simulink model "building_HVAC_V00_027_AI_2019b"  (R2021b)
settings: Solver=ode3  StartTime=1425600  StopTime=1429297  FixedStep=0.1  RelTol=1e-3
model workspace (MAT data in the model file):
  A = 0
  pystep = 1
values from neighbouring files (symbols this model uses):
  Air_Cp = [1007 1007 1006 1006 1006 1006 1006 1006 1006 1006 1007 1007 ... (21 elements, 21x1)]    [data_07.mat]    (also in data_08.mat)
  Air_density = [1.783 1.582 1.422 1.367 1.341 1.316 1.292 1.268 1.246 1.225 1.204 1.184 ... (32 elements, 32x1)]    [data_07.mat]    (also in data_08.mat)
  Air_dynamic_viscosity_PaS = [1.318e-05 1.456e-05 1.588e-05 1.64e-05 1.665e-05 1.69e-05 1.715e-05 1.74e-05 1.764e-05 1.789e-05 1.813e-05 1.837e-05 ... (32 elements, 32x1)]    [data_07.mat]    (also in data_08.mat)
  Air_enthalpy = [325420 335490 345550 355620 365680 375730 385790 395850 405910 415970 426040 436110 ... (21 elements, 21x1)]    [data_07.mat]    (also in data_08.mat)
  Air_prandtl_number = [0.734 0.72 0.711 0.707 0.705 0.701 0.699 0.698 0.699 0.702]    [data_07.mat]    (also in data_08.mat)
  Air_Temp_for_Cp = [200 210 220 230 240 250 260 270 280 290 300 310 ... (21 elements, 21x1)]    [data_07.mat]    (also in data_08.mat)
  Air_Temp_for_density = [-75 -50 -25 -15 -10 -5 0 5 10 15 20 25 ... (32 elements, 32x1)]    [data_07.mat]    (also in data_08.mat)
  Air_Temp_for_dynamic_viscosity = [-75 -50 -25 -15 -10 -5 0 5 10 15 20 25 ... (32 elements, 32x1)]    [data_07.mat]    (also in data_08.mat)
  Air_Temp_for_enthalpy = [200 210 220 230 240 250 260 270 280 290 300 310 ... (21 elements, 21x1)]    [data_07.mat]    (also in data_08.mat)
  Air_Temp_for_prandtl_number = [-100 -50 0 25 50 100 150 200 250 300]    [data_07.mat]    (also in data_08.mat)
  Air_Temp_for_thermal_conductivity = [-190 -150 -100 -75 -50 -25 -15 -10 -5 0 5 10 ... (35 elements, 35x1)]    [data_07.mat]    (also in data_08.mat)
  Air_thermal_conductivity = [0.00782 0.01169 0.0162 0.01834 0.02041 0.02241 0.0232 0.02359 0.02397 0.02436 0.02474 0.02512 ... (35 elements, 35x1)]    [data_07.mat]    (also in data_08.mat)
  Ambient_Solar_heat_Seoul_20200701_to_20200731 = [0 0 0 0 0 0 2.777777778 38.88888889 72.22222222 97.22222222 333.3333333 263.8888889 ... (745 elements, 745x1)]    [data_07.mat]    (also in data_08.mat)
  Ambient_Solar_heat_Seoul_20200701_to_20210630 = [0 0 0 0 0 2.777777778 38.88888889 72.22222222 97.22222222 333.3333333 263.8888889 152.7777778 ... (8736 elements, 8736x1)]    [data_07.mat]    (also in data_08.mat)
  Ambient_Solar_heat_Seoul_20200801_to_20200831 = [0 0 0 0 0 0 2.777777778 11.11111111 38.88888889 63.88888889 127.7777778 258.3333333 ... (745 elements, 745x1)]    [data_07.mat]    (also in data_08.mat)
  Ambient_Solar_heat_Seoul_20200901_to_20200930 = [0 0 0 0 0 0 0 22.22222222 108.3333333 141.6666667 211.1111111 386.1111111 ... (721 elements, 721x1)]    [data_07.mat]    (also in data_08.mat)
  Ambient_Temp_Seoul_20200701_to_20200731 = [18.8 18.8 18.7 18.4 18.2 18.2 18.3 18.5 19.1 19.6 21.2 21.6 ... (745 elements, 745x1)]    [data_07.mat]    (also in data_08.mat)
  Ambient_Temp_Seoul_20200701_to_20210630 = [18.8 18.7 18.4 18.2 18.2 18.3 18.5 19.1 19.6 21.2 21.6 21.7 ... (8736 elements, 8736x1)]    [data_07.mat]    (also in data_08.mat)
  Ambient_Temp_Seoul_20200801_to_20200831 = [25 24.6 24.6 24.7 24.7 24.5 24.3 24.3 24.6 25 25.7 26.8 ... (745 elements, 745x1)]    [data_07.mat]    (also in data_08.mat)
  Ambient_Temp_Seoul_20200901_to_20200930 = [26.2 25.8 25.5 24.9 24.5 24.3 24 23.9 24.4 24.8 25.7 26.6 ... (721 elements, 721x1)]    [data_07.mat]    (also in data_08.mat)
  Ambient_Time_Seoul_20200701_to_20200731 = [0 3600 7200 10800 14400 18000 21600 25200 28800 32400 36000 39600 ... (745 elements, 745x1)]    [data_07.mat]    (also in data_08.mat)
  Ambient_Time_Seoul_20200701_to_20210630 = [0 3600 7200 10800 14400 18000 21600 25200 28800 32400 36000 39600 ... (8736 elements, 8736x1)]    [data_07.mat]    (also in data_08.mat)
  Ambient_Time_Seoul_20200901_to_20200930 = [0 3600 7200 10800 14400 18000 21600 25200 28800 32400 36000 39600 ... (721 elements, 721x1)]    [data_07.mat]    (also in data_08.mat)
  Ambient_Water_Vapor_Pressure_Seoul_20200701_to_20200731 = [18.4 18.8 18.6 18.2 17.9 17.7 18.6 18.6 18.5 19.1 19.9 19.5 ... (745 elements, 745x1)]    [data_07.mat]    (also in data_08.mat)
  Ambient_Water_Vapor_Pressure_Seoul_20200701_to_20210630 = [18.8 18.6 18.2 17.9 17.7 18.6 18.6 18.5 19.1 19.9 19.5 19.4 ... (8736 elements, 8736x1)]    [data_07.mat]    (also in data_08.mat)
  Ambient_Water_Vapor_Pressure_Seoul_20200801_to_20200831 = [28.4 27.7 28.1 28.8 29.1 28.8 28.8 29.1 29.7 30 31.3 29.8 ... (745 elements, 745x1)]    [data_07.mat]    (also in data_08.mat)
  Ambient_Water_Vapor_Pressure_Seoul_20200901_to_20200930 = [26.1 25.8 25.6 24.7 24 24.3 22.9 23.1 23.1 22.8 24 24.3 ... (721 elements, 721x1)]    [data_07.mat]    (also in data_08.mat)
  Ambient_wind_speed_Seoul_20200701_to_20200731 = [3.7 3 3 2.3 1.2 1.5 3.1 1.4 1 1.4 2.5 2.1 ... (745 elements, 745x1)]    [data_07.mat]    (also in data_08.mat)
  Ambient_wind_speed_Seoul_20200701_to_20210630 = [3 3 2.3 1.2 1.5 3.1 1.4 1 1.4 2.5 2.1 2 ... (8736 elements, 8736x1)]    [data_07.mat]    (also in data_08.mat)
  Ambient_wind_speed_Seoul_20200801_to_20200831 = [3.4 0.5 0.5 1.2 0.8 1.3 1.8 1.4 1.2 1.1 1.8 3.4 ... (745 elements, 745x1)]    [data_07.mat]    (also in data_08.mat)
  Ambient_wind_speed_Seoul_20200901_to_20200930 = [2.3 2.2 2.5 2.6 2.4 2.1 1.7 2.7 2.6 2.5 1.5 1.8 ... (721 elements, 721x1)]    [data_07.mat]    (also in data_08.mat)
  init_time = start_time +60    [SIMULINK_RUn.m]    (also in data_07.mat = 0; data_08.mat = 1425660)
  Initial_Temp = 273 + 28    (= 301)    [SIMULINK_RUn.m]    (also in data_07.mat = 285; data_08.mat = 302)
  Shadow_20200701_to_20210630 = [285 300 315 330 345 360 15 30 45 60 75 90 ... (8736 elements, 8736x1)]    [data_07.mat]    (also in data_08.mat)
  start_time = 12 * 3600 + da * day_to_sec    [SIMULINK_RUn.m]    (also in data_07.mat = 0; data_08.mat = 1425600)
  Under_30cm_ground_Temp_Seoul_20200701_to_20200731 = [22.6 22.6 22.5 22.5 22.4 22.3 22.3 22.2 22.1 22.1 22 22 ... (745 elements, 745x1)]    [data_07.mat]    (also in data_08.mat)
  Under_30cm_ground_Temp_Seoul_20200701_to_20210630 = [22.6 22.5 22.5 22.4 22.3 22.3 22.2 22.1 22.1 22 22 22 ... (8736 elements, 8736x1)]    [data_07.mat]    (also in data_08.mat)
  Under_30cm_ground_Temp_Seoul_20200801_to_20200831 = [25.6 25.6 25.6 25.5 25.5 25.5 25.4 25.4 25.3 25.3 25.3 25.2 ... (745 elements, 745x1)]    [data_07.mat]    (also in data_08.mat)
  Under_30cm_ground_Temp_Seoul_20200901_to_20200930 = [27.4 27.4 27.4 27.4 27.3 27.3 27.3 27.2 27.2 27.1 27 27 ... (721 elements, 721x1)]    [data_07.mat]    (also in data_08.mat)
  water_saturation_enthalpy_latent = [2500899.39 2498955.8 2496540.3 2494128 2491818 2489411 2487006 2484604 2482303 2479905 2477508 2475213 ... (64 elements, 64x1)]    [data_07.mat]    (also in data_08.mat)
  water_saturation_enthalpy_vapor = [2500900 2502500 2504300 2506100 2508000 2509800 2511600 2513400 2515300 2517100 2518900 2520800 ... (64 elements, 64x1)]    [data_07.mat]    (also in data_08.mat)
  water_saturation_pressure = [611.65 650.03 698.46 750.07 805.02 863.5 925.7 991.83 1062.2 1136.8 1216 1300 ... (64 elements, 64x1)]    [data_07.mat]    (also in data_08.mat)
  water_Temp_for_saturation_enthalpy_latent = [273.16 274 275 276 277 278 279 280 281 282 283 284 ... (64 elements, 64x1)]    [data_07.mat]    (also in data_08.mat)
  water_Temp_for_saturation_enthalpy_vapor = [273.16 274 275 276 277 278 279 280 281 282 283 284 ... (64 elements, 64x1)]    [data_07.mat]    (also in data_08.mat)
  water_Temp_for_saturation_pressure = [273.16 274 275 276 277 278 279 280 281 282 283 284 ... (64 elements, 64x1)]    [data_07.mat]    (also in data_08.mat)
undefined symbols (not defined in the file or in its folder): DiscIntNeverNeededParam
libraries: fuzblock x1
(part 1 of 3)
settings Model: SimulationMode=accelerator  Creator=HYUNJONG OH  LastModifiedBy=b811043
settings SolverCC: AlgebraicLoopSolver=TrustRegion  AutoInsertRateTranBlk=on
settings DataIOCC: ExternalInput=[0,input_total(1),input_total(2),input_total(3),input_total(4),input_total(5),input_total(6);(24*3600),input_total(1),input_total(2),input_total(3),input_total(4),input_total(5),input_total(6)]  SaveFormat=Array  SaveOutput=off  SaveTime=off
settings DebuggingCC: AlgebraicLoopMsg=none  SFMachineParentedDataDiag=warning  ArithmeticOperatorsInVariantConditions=warning
settings SFSimCC: CustomCodeUndefinedFunction=UseInterfaceOnly

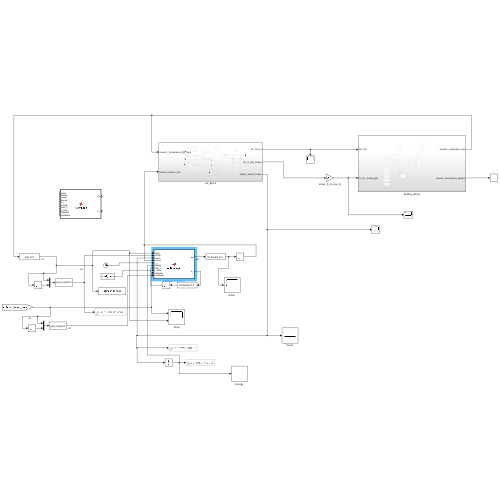
[thumbnail: Simulink's stored preview of the top-level diagram]
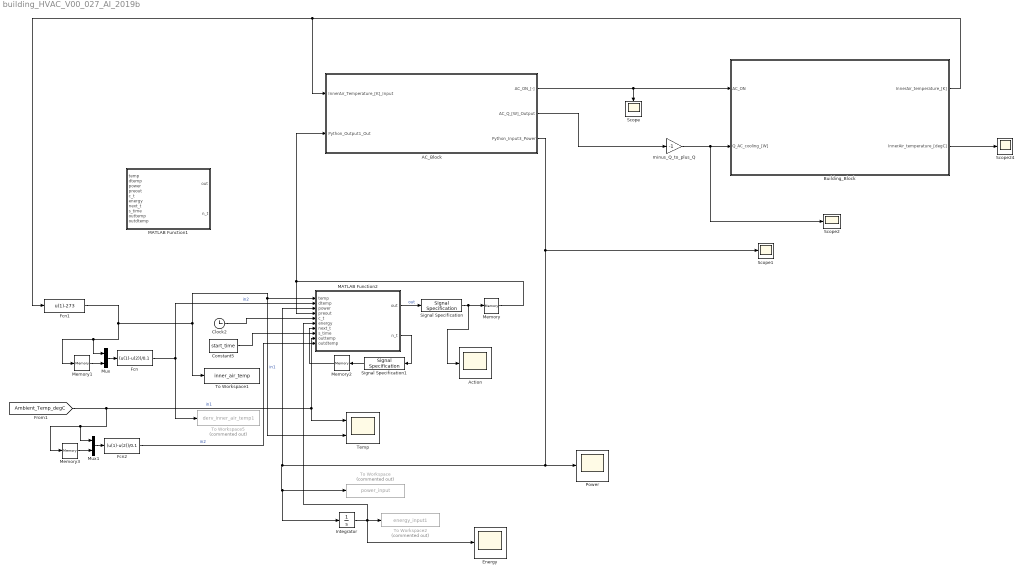
== system building_HVAC_V00_027_AI_2019b ==
  AC_Block : Subsystem
  Action : Scope
  Building_Block : Subsystem
  Clock2 : Clock
  Constant5 : Constant  Value=start_time
  Energy : Scope
  Fcn : Fcn  Expr=(u(1)-u(2))/0.1
  Fcn1 : Fcn  Expr=u(1)-273
  Fcn2 : Fcn  Expr=(u(1)-u(2))/0.1
  Integrator : Integrator
  MATLAB Function1 : MATLAB Function
  MATLAB Function2 : MATLAB Function
  Memory : Memory  InheritSampleTime=on
  Memory1 : Memory  InitialCondition=301 - 273  InheritSampleTime=on
  Memory2 : Memory  InitialCondition=init_time  InheritSampleTime=on
  Memory3 : Memory  InitialCondition=301 - 273  InheritSampleTime=on
  Mux : Mux  Inputs=2
  Mux1 : Mux  Inputs=2
  Power : Scope
  Scope{,1..2,24} (4 alike) : Scope
  Signal Specification : SignalSpecification  OutDataTypeStr=double  Dimensions=1
  Signal Specification1 : SignalSpecification  OutDataTypeStr=double  Dimensions=1
  Temp : Scope  NumInputPorts=2
  To Workspace : ToWorkspace  Commented=on  VariableName=power_input  SampleTime=-1
      settings: Save2DSignal=2-D array (concatenate along first dimension)
  To Workspace1 : ToWorkspace  VariableName=inner_air_temp  SampleTime=-1
      settings: Decimation=10  Save2DSignal=2-D array (concatenate along first dimension)
  To Workspace2 : ToWorkspace  Commented=on  VariableName=energy_input1  SampleTime=-1
      settings: Save2DSignal=2-D array (concatenate along first dimension)
  To Workspace5 : ToWorkspace  Commented=on  VariableName=derv_inner_air_temp1  SampleTime=-1
      settings: Save2DSignal=2-D array (concatenate along first dimension)
  minus_Q_to_plus_Q : Gain  Gain=-1
  wires:
  Fcn1/1 -> Memory1/1, Mux/1, MATLAB Function2/1(temp), Temp/2, To Workspace1/1  "in1"
  Fcn/1 -> MATLAB Function2/2(dtemp), To Workspace5/1  "in2"
  Mux/1 -> Fcn/1
  Memory1/1 -> Mux/2
  MATLAB Function2/1(out) -> Signal Specification/1  "out"
  Clock2/1 -> MATLAB Function2/5(c_t)
  Integrator/1 -> MATLAB Function2/6(energy), To Workspace2/1, Energy/1
  MATLAB Function2/2(n_t) -> Signal Specification1/1
  Signal Specification1/1 -> Memory2/1
  Memory2/1 -> MATLAB Function2/7(next_t)
  Constant5/1 -> MATLAB Function2/8(s_time)
  Signal Specification/1 -> Memory/1, Action/1
  AC_Block/3(Python_Input3_Power) -> Scope1/1, MATLAB Function2/3(power), Integrator/1, To Workspace/1, Power/1
  AC_Block/2(AC_Q_[W]_Output) -> minus_Q_to_plus_Q/1
  AC_Block/1(AC_ON_[-]) -> Building_Block/1(AC_ON), Scope/1
  Building_Block/1(InnerAir_temperature_[K]) -> Fcn1/1, AC_Block/1(InnerAir_Temperature_[K]_Input)
  Building_Block/2(InnerAir_temperature_[degC]) -> Scope24/1
  minus_Q_to_plus_Q/1 -> Scope2/1, Building_Block/2(Q_AC_cooling_[W])
  Memory/1 -> MATLAB Function2/4(preout), AC_Block/2(Python_Output1_Out)
  Memory3/1 -> Mux1/2
  Fcn2/1 -> MATLAB Function2/10(outdtemp)  "in2"
  Mux1/1 -> Fcn2/1
  [Ambient_Temp_degC] -> Memory3/1, Mux1/1, MATLAB Function2/9(outtemp), Temp/1  "in1"

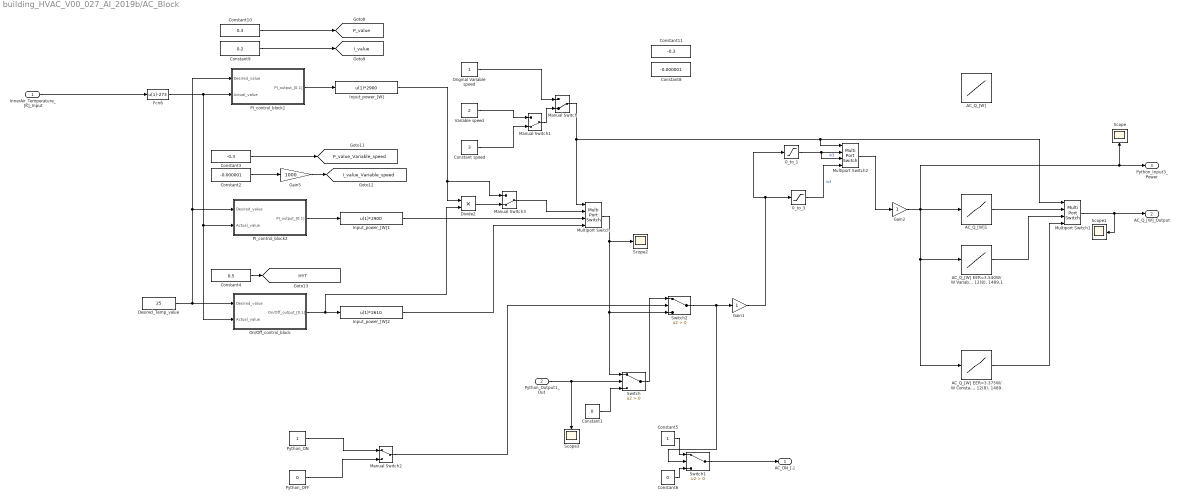
== system building_HVAC_V00_027_AI_2019b/AC_Block ==
  InnerAir_Temperature_[K]_Input : Inport
  Python_Output1_Out : Inport  Port=2
  0_to_1 : Saturate  UpperLimit=2900  LowerLimit=0
  0_to_3 : Saturate  UpperLimit=2610  LowerLimit=0
  AC_Q_[W] : Lookup_n-D  NumberOfTableDimensions=1  BreakpointsForDimension1=[0;2000]  Table=[0;((-1)*2000*3.0)]  InternalRulePriority=Speed  RndMeth=Simplest  InputSameDT=on
  "AC_Q_[W] EER=3.375W/W Constant sped type compressor is used thus, the control strategy must be ON/OFF control method Lim, J., Yoon, M. S., Al-Qahtani, T., & Nam, Y. (2019). Feasibility study on variable-speed air conditioner under hot climate based on real-scale experiment and energy simulation. Energies, 12(8), 1489." : Lookup_n-D  NumberOfTableDimensions=1  BreakpointsForDimension1=[0;2610]  Table=[0;((-1)*2610*3.375)]  InternalRulePriority=Speed  RndMeth=Simplest  InputSameDT=on
  "AC_Q_[W] EER=3.540W/W Variable sped type compressor is used thus, the control strategy should be part-load control method Lim, J., Yoon, M. S., Al-Qahtani, T., & Nam, Y. (2019). Feasibility study on variable-speed air conditioner under hot climate based on real-scale experiment and energy simulation. Energies, 12(8), 1489.1" : Lookup_n-D  NumberOfTableDimensions=1  BreakpointsForDimension1=[0;2900]  Table=[0;((-1)*2900*3.540)]  InternalRulePriority=Speed  RndMeth=Simplest  InputSameDT=on
  AC_Q_[W]1 : Lookup_n-D  NumberOfTableDimensions=1  BreakpointsForDimension1=[0;2900]  Table=[0;((-1)*2900*3.7143)]  InternalRulePriority=Speed  RndMeth=Simplest  InputSameDT=on
  Constant speed : Constant  Value=3
  Constant1 : Constant  Value=0
  Constant10 : Constant  Value=0.3
  Constant11 : Constant  Value=-0.3
  Constant2 : Constant  Value=-0.000001
  Constant3 : Constant  Value=-0.3
  Constant4 : Constant  Value=0.5
  Constant5 : Constant
  Constant6 : Constant  Value=0
  Constant8 : Constant  Value=-0.000001
  Constant9 : Constant  Value=0.2
  Desired_Temp_value : Constant  Value=25
  Divide2 : Product  Inputs=**
  Fcn6 : Fcn  Expr=u(1)-273
  Gain1 : Gain
  Gain2 : Gain
  Gain5 : Gain  Gain=1000
  Input_power_[W] : Fcn  Expr=u(1)*2900
  Input_power_[W]1 : Fcn  Expr=u(1)*2900
  Input_power_[W]2 : Fcn  Expr=u(1)*2610
  Manual Switch : ManualSwitch  CurrentSetting=0
  Manual Switch1 : ManualSwitch  CurrentSetting=0
  Manual Switch2 : ManualSwitch
  Manual Switch3 : ManualSwitch  CurrentSetting=0
  Multiport Switch : MultiPortSwitch
  Multiport Switch1 : MultiPortSwitch
  Multiport Switch2 : MultiPortSwitch
  On/Off_control_block : Subsystem
  Original Variable speed : Constant
  PI_control_block1 : Subsystem
  PI_control_block2 : Subsystem
  Python_OFF : Constant  Value=0
  Python_ON : Constant
  Scope{,1..3} (4 alike) : Scope
  Switch : Switch  Criteria=u2 > Threshold
  Switch1 : Switch  Criteria=u2 > Threshold
  Switch2 : Switch  Criteria=u2 > Threshold
  Variable speed : Constant  Value=2
  AC_ON_[-] : Outport
  AC_Q_[W]_Output : Outport  Port=2
  Python_Input3_Power : Outport  Port=3
  tag scope: HYT=global, I_value=global, I_value_Variable_speed=global, P_value=global, P_value_Variable_speed=global
  wires:
  Python_Output1_Out/1 -> Switch/2, Scope3/1
  Manual Switch/1 -> Multiport Switch1/1, Multiport Switch2/1, Multiport Switch/1
  Desired_Temp_value/1 -> PI_control_block1/1(Desired_value), PI_control_block2/1(Desired_value), On/Off_control_block/1(Desired_value)
  Fcn6/1 -> On/Off_control_block/2(Actual_value), PI_control_block2/2(Actual_value), PI_control_block1/2(Actual_value)
  InnerAir_Temperature_[K]_Input/1 -> Fcn6/1
  PI_control_block2/1(PI_output_[0,1]) -> Input_power_[W]1/1
  Constant1/1 -> Switch/3
  Constant4/1 -> [HYT]
  Original Variable speed/1 -> Manual Switch/1
  Manual Switch1/1 -> Manual Switch/2
  Constant speed/1 -> Manual Switch1/2
  Input_power_[W]1/1 -> Multiport Switch/3
  Input_power_[W]2/1 -> Multiport Switch/4
  Multiport Switch2/1 -> Gain2/1
  AC_Q_[W]1/1 -> Multiport Switch1/2
  0_to_1/1 -> Multiport Switch2/3, Multiport Switch2/2  "in3"
  PI_control_block1/1(PI_output_[0,1]) -> Input_power_[W]/1
  Variable speed/1 -> Manual Switch1/1
  On/Off_control_block/1(On/Off_output_[0,1]) -> Divide2/2, Input_power_[W]2/1
  0_to_3/1 -> Multiport Switch2/4  "in3"
  Gain2/1 -> AC_Q_[W]1/1, "AC_Q_[W] EER=3.375W/W Constant sped type compressor is used thus, the control strategy must be ON/OFF control method Lim, J., Yoon, M. S., Al-Qahtani, T., & Nam, Y. (2019). Feasibility study on variable-speed air conditioner under hot climate based on real-scale experiment and energy simulation. Energies, 12(8), 1489."/1, "AC_Q_[W] EER=3.540W/W Variable sped type compressor is used thus, the control strategy should be part-load control method Lim, J., Yoon, M. S., Al-Qahtani, T., & Nam, Y. (2019). Feasibility study on variable-speed air conditioner under hot climate based on real-scale experiment and energy simulation. Energies, 12(8), 1489.1"/1, Python_Input3_Power/1, Scope/1
  Multiport Switch1/1 -> Scope1/1, AC_Q_[W]_Output/1
  Constant5/1 -> Switch1/1
  Constant6/1 -> Switch1/3
  Gain1/1 -> 0_to_1/1, 0_to_3/1
  Multiport Switch/1 -> Scope2/1, Switch2/3, Switch/1
  Switch1/1 -> AC_ON_[-]/1
  Python_OFF/1 -> Manual Switch2/2
  Python_ON/1 -> Manual Switch2/1
  Manual Switch2/1 -> Switch2/2
  Switch/1 -> Switch2/1
  Switch2/1 -> Switch1/2, Gain1/1
  "AC_Q_[W] EER=3.540W/W Variable sped type compressor is used thus, the control strategy should be part-load control method Lim, J., Yoon, M. S., Al-Qahtani, T., & Nam, Y. (2019). Feasibility study on variable-speed air conditioner under hot climate based on real-scale experiment and energy simulation. Energies, 12(8), 1489.1"/1 -> Multiport Switch1/3
  "AC_Q_[W] EER=3.375W/W Constant sped type compressor is used thus, the control strategy must be ON/OFF control method Lim, J., Yoon, M. S., Al-Qahtani, T., & Nam, Y. (2019). Feasibility study on variable-speed air conditioner under hot climate based on real-scale experiment and energy simulation. Energies, 12(8), 1489."/1 -> Multiport Switch1/4
  Constant2/1 -> Gain5/1
  Constant3/1 -> [P_value_Variable_speed]
  Gain5/1 -> [I_value_Variable_speed]
  Input_power_[W]/1 -> Manual Switch3/1, Divide2/1
  Divide2/1 -> Manual Switch3/2
  Manual Switch3/1 -> Multiport Switch/2
  Constant9/1 -> [I_value]
  Constant10/1 -> [P_value]

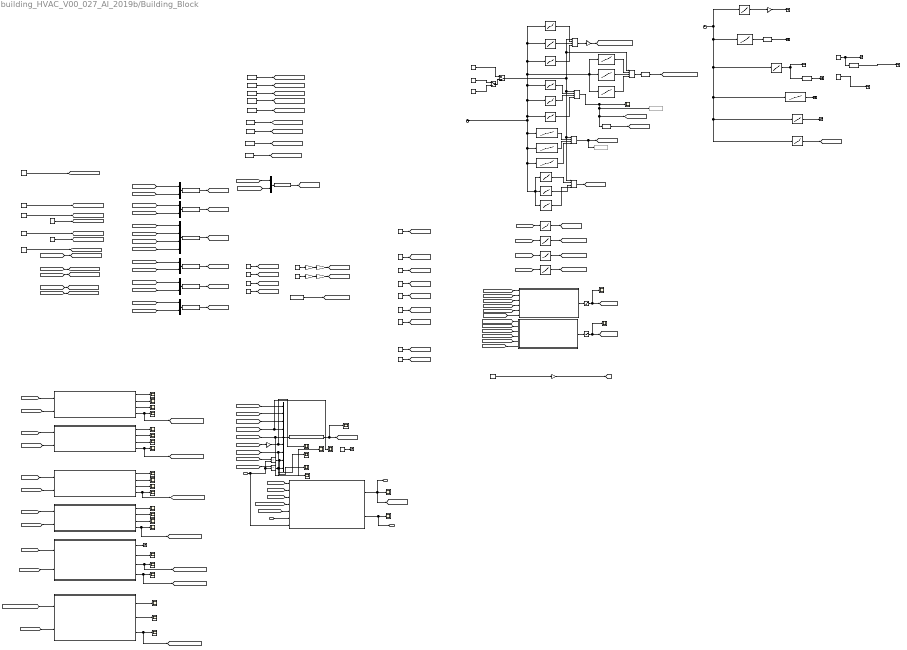
== system building_HVAC_V00_027_AI_2019b/Building_Block ==
  AC_ON : Inport
  Q_AC_cooling_[W] : Inport  Port=2
  20200701_to_20200731 : Constant
  20200801_to_20200831 : Constant  Value=2
  20200901_to_20200930 : Constant  Value=3
  A=Area_East : Fcn  Expr=u(1)*u(2)
  A=Area_North : Fcn  Expr=u(1)*u(2)
  A=Area_South - Area_Window2 : Fcn  Expr=u(1)*u(2)-u(3)*u(4)
  A=Area_West : Fcn  Expr=u(1)*u(2)
  A=Area_floor : Fcn  Expr=u(1)*u(2)
  A=Area_window : Fcn  Expr=u(1)*u(2)
  AC_blower_Volume_flow_rate_[m3/s] : Constant  Value=0.2*0.5*0.5
  AC_evaporator_vertical_length_[m] : Constant  Value=0.5
  Air_Prandtl_number_(-) _of_Air_temperature_(degC) : Lookup_n-D  NumberOfTableDimensions=1  BreakpointsForDimension1=Air_Temp_for_prandtl_number  Table=Air_prandtl_number  InternalRulePriority=Speed  RndMeth=Simplest  InputSameDT=on
  Air_Thermal_conductivity_(W/mK) _of_Air_temperature_(degC) : Lookup_n-D  NumberOfTableDimensions=1  BreakpointsForDimension1=Air_Temp_for_thermal_conductivity  Table=Air_thermal_conductivity  InternalRulePriority=Speed  RndMeth=Simplest  InputSameDT=on
  Air_density_(kg/m3) _of_Air_temperature_(degC) : Lookup_n-D  NumberOfTableDimensions=1  BreakpointsForDimension1=Air_Temp_for_density  Table=Air_density  InternalRulePriority=Speed  RndMeth=Simplest  InputSameDT=on
  Air_dynamic_viscosity_(Pa s) _of_Air_temperature_(degC) : Lookup_n-D  NumberOfTableDimensions=1  BreakpointsForDimension1=Air_Temp_for_dynamic_viscosity  Table=Air_dynamic_viscosity_PaS  InternalRulePriority=Speed  RndMeth=Simplest  InputSameDT=on
  Air_wind_speed_(m/s) _of_Air_temperature_(degC)08 : Lookup_n-D  NumberOfTableDimensions=1  BreakpointsForDimension1=Ambient_Time_Seoul_20200701_to_20200731  Table=Ambient_wind_speed_Seoul_20200801_to_20200831  InternalRulePriority=Speed  RndMeth=Simplest  InputSameDT=on
  Air_wind_speed_(m/s) _of_Air_temperature_(degC)09 : Lookup_n-D  NumberOfTableDimensions=1  BreakpointsForDimension1=Ambient_Time_Seoul_20200901_to_20200930  Table=Ambient_wind_speed_Seoul_20200901_to_20200930  InternalRulePriority=Speed  RndMeth=Simplest  InputSameDT=on
  Air_wind_speed_(m/s) _of_Air_temperature_(degC)1 : Lookup_n-D  NumberOfTableDimensions=1  BreakpointsForDimension1=Ambient_Time_Seoul_20200701_to_20210630  Table=Ambient_wind_speed_Seoul_20200701_to_20210630  InternalRulePriority=Speed  RndMeth=Simplest  InputSameDT=on
  Air_wind_speed_(m/s) _of_Time : Lookup_n-D  NumberOfTableDimensions=1  BreakpointsForDimension1=Ambient_Time_Seoul_20200701_to_20200731  Table=Ambient_wind_speed_Seoul_20200701_to_20200731  InternalRulePriority=Speed  RndMeth=Simplest  InputSameDT=on
  Ambient_Temp_K1 : Terminator
  Ambient_Temp_K2 : Terminator
  Ambient_Temp_degC1 : Terminator
  Ambient_Temp_degC2 : Terminator
  Ambient_Water_Vapor_Pressure : Terminator
  Blower_and_InnerAir_Block : Subsystem
  Clock : Clock
  Clock1 : Clock
  Constant : Constant  Value=0.1
  Constant{1..5} (5 alike) : Constant  Value=0.2
  Constant6 : Constant  Value=35
  Constant7 : Constant  Value=500
  Constant8 : Constant  Value=4500
  "Cp_cement Masonry Materials Cement mortar Frank P. Incropera and David P. DeWitt, \"Fundamentals of Heat and Mass Transfer\", (1996), FOURTH EDITION, pg. 833" : Constant  Value=780
  "Cp_insulator Board and Slab Cellular glass Frank P. Incropera and David P. DeWitt, \"Fundamentals of Heat and Mass Transfer\", (1996), FOURTH EDITION, pg. 834" : Constant  Value=1000
  Cp_window : Constant  Value=840
  East_Wall_Block : Subsystem
  East_Wall_horizontal_length_[m]3 : Constant  Value=8
  Fcn{1..5} (5 alike) : Fcn  Expr=u(1)+273
  Floorl_Block : Subsystem
  Gain : Gain
  Gain1 : Gain  Gain=0.1
  Infiltration_[L/hr] : Constant  Value=0.4
  Initial_InnerAir_Temp_[K] : Constant  Value=Initial_Temp  VectorParams1D=off
  InnerWall_Depth : Constant  Value=0.15
  "Inside_convection_heat_coefficient_H_(summer) [Kreider J. F. et al., pp.264] [Kreider, J. F., Curtiss, P. S., & Rabl, A. (2009). Heating and cooling of buildings: design for efficiency. CRC Press.]" : Constant  Value=22.7
  Insulator_Depth : Constant  Value=0.15
  Manual Switch1 : ManualSwitch  CurrentSetting=0
  Manual Switch2 : ManualSwitch
  Multiport Switch{,1..4} (5 alike) : MultiPortSwitch
  Mux{1,3,5..8} (6 alike) : Mux  Inputs=2
  Mux2 : Mux
  Mux4 : Mux  Inputs=9
  North_Wall_Block : Subsystem
  OuterWall_Depth : Constant  Value=0.15
  Product : Product
  Product1 : Product
  Q_total_to_InnerAir1 : Terminator
  Q_total_to_InnerAir_[W] : Fcn  Expr=u(1)+u(2)+u(3)+u(4)+u(5)+u(6)+u(7)+u(8)-u(9)
  Saturation : Saturate  UpperLimit=inf  LowerLimit=0.000001
  Saturation1 : Saturate  UpperLimit=inf  LowerLimit=0.000001
  Scope{,1..33} (34 alike) : Scope
  Seoul_Seoul_Temp_(degC) 20200701_to_1 : Lookup_n-D  NumberOfTableDimensions=1  BreakpointsForDimension1=Ambient_Time_Seoul_20200701_to_20210630  Table=Ambient_Temp_Seoul_20200701_to_20210630  InternalRulePriority=Speed  RndMeth=Simplest  InputSameDT=on
  Seoul_Seoul_Temp_(degC) 20200701_to_20200731 : Lookup_n-D  NumberOfTableDimensions=1  BreakpointsForDimension1=Ambient_Time_Seoul_20200701_to_20200731  Table=Ambient_Temp_Seoul_20200701_to_20200731  InternalRulePriority=Speed  RndMeth=Simplest  InputSameDT=on
  Seoul_Seoul_Temp_(degC) 20200801_to_20200831 : Lookup_n-D  NumberOfTableDimensions=1  BreakpointsForDimension1=Ambient_Time_Seoul_20200701_to_20200731  Table=Ambient_Temp_Seoul_20200801_to_20200831  InternalRulePriority=Speed  RndMeth=Simplest  InputSameDT=on
  Seoul_Seoul_Temp_(degC) 20200901_to_20200930 : Lookup_n-D  NumberOfTableDimensions=1  BreakpointsForDimension1=Ambient_Time_Seoul_20200901_to_20200930  Table=Ambient_Temp_Seoul_20200901_to_20200930  InternalRulePriority=Speed  RndMeth=Simplest  InputSameDT=on
  Seoul_Solar_heat_flux_(W/m2) 20200701_to_1 : Lookup_n-D  NumberOfTableDimensions=1  BreakpointsForDimension1=Ambient_Time_Seoul_20200701_to_20210630  Table=Ambient_Solar_heat_Seoul_20200701_to_20210630  InternalRulePriority=Speed  RndMeth=Simplest  InputSameDT=on
  Seoul_Solar_heat_flux_(W/m2) 20200701_to_20200731 : Lookup_n-D  NumberOfTableDimensions=1  BreakpointsForDimension1=Ambient_Time_Seoul_20200701_to_20200731  Table=Ambient_Solar_heat_Seoul_20200701_to_20200731  InternalRulePriority=Speed  RndMeth=Simplest  InputSameDT=on
  Seoul_Solar_heat_flux_(W/m2) 20200801_to_20200831 : Lookup_n-D  NumberOfTableDimensions=1  BreakpointsForDimension1=Ambient_Time_Seoul_20200701_to_20200731  Table=Ambient_Solar_heat_Seoul_20200801_to_20200831  InternalRulePriority=Speed  RndMeth=Simplest  InputSameDT=on
  Seoul_Solar_heat_flux_(W/m2) 20200901_to_20200930 : Lookup_n-D  NumberOfTableDimensions=1  BreakpointsForDimension1=Ambient_Time_Seoul_20200901_to_20200930  Table=Ambient_Solar_heat_Seoul_20200901_to_20200930  InternalRulePriority=Speed  RndMeth=Simplest  InputSameDT=on
  Seoul_ambient_water_vapor_pressure_(hPa) 20200701_to_1 : Lookup_n-D  NumberOfTableDimensions=1  BreakpointsForDimension1=Ambient_Time_Seoul_20200701_to_20210630  Table=Ambient_Water_Vapor_Pressure_Seoul_20200701_to_20210630  InternalRulePriority=Speed  RndMeth=Simplest  InputSameDT=on
  Seoul_ambient_water_vapor_pressure_(hPa) 20200701_to_20200731 : Lookup_n-D  NumberOfTableDimensions=1  BreakpointsForDimension1=Ambient_Time_Seoul_20200701_to_20200731  Table=Ambient_Water_Vapor_Pressure_Seoul_20200701_to_20200731  InternalRulePriority=Speed  RndMeth=Simplest  InputSameDT=on
  Seoul_ambient_water_vapor_pressure_(hPa) 20200801_to_20200831 : Lookup_n-D  NumberOfTableDimensions=1  BreakpointsForDimension1=Ambient_Time_Seoul_20200701_to_20200731  Table=Ambient_Water_Vapor_Pressure_Seoul_20200801_to_20200831  InternalRulePriority=Speed  RndMeth=Simplest  InputSameDT=on
  Seoul_ambient_water_vapor_pressure_(hPa) 20200901_to_20200930 : Lookup_n-D  NumberOfTableDimensions=1  BreakpointsForDimension1=Ambient_Time_Seoul_20200901_to_20200930  Table=Ambient_Water_Vapor_Pressure_Seoul_20200901_to_20200930  InternalRulePriority=Speed  RndMeth=Simplest  InputSameDT=on
  Seoul_under_30cm_ground_temperature_(degC) 20200701_to_1 : Lookup_n-D  NumberOfTableDimensions=1  BreakpointsForDimension1=Ambient_Time_Seoul_20200701_to_20210630  Table=Under_30cm_ground_Temp_Seoul_20200701_to_20210630  InternalRulePriority=Speed  RndMeth=Simplest  InputSameDT=on
  Seoul_under_30cm_ground_temperature_(degC) 20200701_to_20200731 : Lookup_n-D  NumberOfTableDimensions=1  BreakpointsForDimension1=Ambient_Time_Seoul_20200701_to_20200731  Table=Under_30cm_ground_Temp_Seoul_20200701_to_20200731  InternalRulePriority=Speed  RndMeth=Simplest  InputSameDT=on
  Seoul_under_30cm_ground_temperature_(degC) 20200801_to_20200831 : Lookup_n-D  NumberOfTableDimensions=1  BreakpointsForDimension1=Ambient_Time_Seoul_20200701_to_20200731  Table=Under_30cm_ground_Temp_Seoul_20200801_to_20200831  InternalRulePriority=Speed  RndMeth=Simplest  InputSameDT=on
  Seoul_under_30cm_ground_temperature_(degC) 20200901_to_20200930 : Lookup_n-D  NumberOfTableDimensions=1  BreakpointsForDimension1=Ambient_Time_Seoul_20200901_to_20200930  Table=Under_30cm_ground_Temp_Seoul_20200901_to_20200930  InternalRulePriority=Speed  RndMeth=Simplest  InputSameDT=on
  Shadow(-) _of_Time(s) : Lookup_n-D  NumberOfTableDimensions=1  BreakpointsForDimension1=Ambient_Time_Seoul_20200701_to_20210630  Table=Shadow_20200701_to_20210630  InternalRulePriority=Speed  RndMeth=Simplest  InputSameDT=on
  South_Wall_Block : Subsystem
  South_Wall_horizontal_length_[m] : Constant  Value=10
  South_Wall_vertical_length_[m] : Constant  Value=2.5
  Subsystem : Subsystem
  Subsystem1 : Subsystem
  Terminator : Terminator
  To Workspace : ToWorkspace  Commented=on  VariableName=outdoor_temp  SampleTime=-1
      settings: Decimation=10  Save2DSignal=2-D array (concatenate along first dimension)
  To Workspace1 : ToWorkspace  Commented=on  VariableName=solar_heat  SampleTime=-1
      settings: Decimation=10  Save2DSignal=2-D array (concatenate along first dimension)
  Under_30cm_soil_Depth_[m] : Constant  Value=0.3
  Under_30cm_soil_temperature_K : Terminator
  Ventilation_[L/hr] : Constant  Value=0.6
  Volume : Fcn  Expr=u(1)*u(2)
  West_Wall_Block : Subsystem
  Wind_Speed : Terminator
  Window_Block : Subsystem
  Window_horizontal_length_[m]66 : Constant  Value=7.5
  Window_vertical_length_[m]66 : Constant  Value=2
  "[1/hr] to [1/s]" : Gain  Gain=1/3600
  "[1/hr] to [1/s]2" : Gain  Gain=1/3600
  "[L] to [m3]" : Gain  Gain=1/1000
  "[L] to [m3]2" : Gain  Gain=1/1000
  "[hPa] to [Pa]" : Gain  Gain=100
  "[hPa] to [Pa]1" : Gain  Gain=100
  "density_cement Masonry Materials Cement mortar Frank P. Incropera and David P. DeWitt, \"Fundamentals of Heat and Mass Transfer\", (1996), FOURTH EDITION, pg. 833" : Constant  Value=1860
  "density_insulator Board and Slab Cellular glass Frank P. Incropera and David P. DeWitt, \"Fundamentals of Heat and Mass Transfer\", (1996), FOURTH EDITION, pg. 834" : Constant  Value=145
  density_window : Constant  Value=2500
  "k_cement Masonry Materials Cement mortar Frank P. Incropera and David P. DeWitt, \"Fundamentals of Heat and Mass Transfer\", (1996), FOURTH EDITION, pg. 833" : Constant  Value=0.72
  "k_insulator Board and Slab Cellular glass Frank P. Incropera and David P. DeWitt, \"Fundamentals of Heat and Mass Transfer\", (1996), FOURTH EDITION, pg. 834" : Constant  Value=0.058
  "k_soil Soil Frank P. Incropera and David P. DeWitt, \"Fundamentals of Heat and Mass Transfer\", (1996), FOURTH EDITION, pg. 838" : Constant  Value=0.52
  solar_heat_flux1 : Terminator
  solar_heat_flux2 : Terminator
  window_absorptivity_[-] : Constant  Value=0.1
  window_depth_[m] : Constant  Value=0.02
  window_transmitivity_[-] : Constant  Value=0.1
  InnerAir_temperature_[K] : Outport
  InnerAir_temperature_[degC] : Outport  Port=2
  tag scope: Ambient_Temp_K=global, Ambient_Temp_degC=global, Ambient_Water_Vapor_Pressure=global, Ambient_air_Prandtl_number=global, Ambient_air_density=global, Ambient_air_dynamic_viscosity=global, Ambient_air_thermal_conductivity=global, Area_East=global, Area_North=global, Area_South=global, Area_West=global, Area_floor=global, Area_window=global, Blower_Volume_Flow_Rate=global, Cp_cement=global, Cp_insulator=global, Cp_window=global, Horizontal_Length_East=global, Horizontal_Length_North=global, Horizontal_Length_South=global, Horizontal_Length_West=global, Horizontal_Length_Window=global, Infiltration=global, Initial_inner_air_Temp=global, InnerAir_Temperature=global, InnerWall_Depth=global, Inside=global, Insulator_Depth=global, OuterWall_Depth=global, Outside_East_West=global, Outside_South_North=global, Q_East_InnerWall_to_InnerAir=global, Q_North_InnerWall_to_InnerAir=global, Q_South_InnerWall_to_InnerAir=global, Q_West_InnerWall_to_InnerAir=global, Q_Window_to_InnerAir=global, Q_floor_to_InnerAir=global, Q_solar_to_InnerAir=global, Q_total_to_InnerAir=global, Under_30cm_soil_Depth=global, Under_30cm_soil_temperature_K=global, Ventilation=global, Vertical_Length_AC_evaporator=global, Vertical_Length_East=global, Vertical_Length_North=global, Vertical_Length_South=global, Vertical_Length_West=global, Vertical_Length_Window=global, Volume_room=global, Wind_Speed=global, absoptivity_wall=global, absorptivity_inner_floor=global, absorptivity_inner_wall_East=global, absorptivity_inner_wall_North=global, absorptivity_inner_wall_South=global, absorptivity_inner_wall_West=global, absorptivity_window=global, density_cement=global, density_insulator=global, density_window=global, k_cement=global, k_insulator=global, k_soil=global, solar_angle_East_to_West=global, solar_heat_flux=global, transmitivity_window=global, window_Depth=global
  wires:
  Mux8/1 -> A=Area_East/1
  A=Area_East/1 -> [Area_East]
  "k_insulator Board and Slab Cellular glass Frank P. Incropera and David P. DeWitt, \"Fundamentals of Heat and Mass Transfer\", (1996), FOURTH EDITION, pg. 834"/1 -> [k_insulator]
  "k_cement Masonry Materials Cement mortar Frank P. Incropera and David P. DeWitt, \"Fundamentals of Heat and Mass Transfer\", (1996), FOURTH EDITION, pg. 833"/1 -> [k_cement]
  OuterWall_Depth/1 -> [OuterWall_Depth]
  Insulator_Depth/1 -> [Insulator_Depth]
  InnerWall_Depth/1 -> [InnerWall_Depth]
  "Cp_insulator Board and Slab Cellular glass Frank P. Incropera and David P. DeWitt, \"Fundamentals of Heat and Mass Transfer\", (1996), FOURTH EDITION, pg. 834"/1 -> [Cp_insulator]
  "Cp_cement Masonry Materials Cement mortar Frank P. Incropera and David P. DeWitt, \"Fundamentals of Heat and Mass Transfer\", (1996), FOURTH EDITION, pg. 833"/1 -> [Cp_cement]
  "density_cement Masonry Materials Cement mortar Frank P. Incropera and David P. DeWitt, \"Fundamentals of Heat and Mass Transfer\", (1996), FOURTH EDITION, pg. 833"/1 -> [density_cement]
  "density_insulator Board and Slab Cellular glass Frank P. Incropera and David P. DeWitt, \"Fundamentals of Heat and Mass Transfer\", (1996), FOURTH EDITION, pg. 834"/1 -> [density_insulator]
  Mux2/1 -> A=Area_South - Area_Window2/1
  [Vertical_Length_South] -> Mux2/2
  [Horizontal_Length_South] -> Mux2/1
  [Horizontal_Length_Window] -> Mux2/3
  [Vertical_Length_Window] -> Mux2/4
  A=Area_South - Area_Window2/1 -> [Area_South]
  South_Wall_vertical_length_[m]/1 -> [Vertical_Length_South]
  East_Wall_horizontal_length_[m]3/1 -> [Horizontal_Length_East]
  South_Wall_horizontal_length_[m]/1 -> [Horizontal_Length_South]
  [Vertical_Length_South] -> [Vertical_Length_East]
  [Vertical_Length_South] -> [Vertical_Length_West]
  [Vertical_Length_South] -> [Vertical_Length_North]
  [Horizontal_Length_South] -> [Horizontal_Length_North]
  [Horizontal_Length_East] -> [Horizontal_Length_West]
  Window_vertical_length_[m]66/1 -> [Vertical_Length_Window]
  Window_horizontal_length_[m]66/1 -> [Horizontal_Length_Window]
  [Horizontal_Length_East] -> Mux8/1
  [Vertical_Length_East] -> Mux8/2
  [Vertical_Length_North] -> Mux1/2
  [Horizontal_Length_North] -> Mux1/1
  A=Area_North/1 -> [Area_North]
  Mux1/1 -> A=Area_North/1
  Mux3/1 -> A=Area_West/1
  [Horizontal_Length_West] -> Mux3/1
  [Vertical_Length_West] -> Mux3/2
  A=Area_West/1 -> [Area_West]
  East_Wall_Block/1(East_outer_concrete_wall_temperature_[degC]) -> Scope/1
  East_Wall_Block/2(East_insulator_temperature_[degC]) -> Scope1/1
  East_Wall_Block/3(East_inner_concrete_wall_temperature_[degC]) -> Scope2/1
  East_Wall_Block/4(Q_East_InnerWall_to_InnerAir_[W]) -> [Q_East_InnerWall_to_InnerAir], Scope3/1
  Air_Prandtl_number_(-) _of_Air_temperature_(degC)/1 -> [Ambient_air_Prandtl_number]
  Subsystem1/1(h (W/(m2)K)) -> Saturation1/1
  Air_dynamic_viscosity_(Pa s) _of_Air_temperature_(degC)/1 -> [Ambient_air_dynamic_viscosity]
  Saturation/1 -> Scope4/1, [Outside_South_North]
  Subsystem/1(h (W/(m2)K)) -> Saturation/1
  Air_Thermal_conductivity_(W/mK) _of_Air_temperature_(degC)/1 -> [Ambient_air_thermal_conductivity]
  Air_density_(kg/m3) _of_Air_temperature_(degC)/1 -> [Ambient_air_density]
  Saturation1/1 -> Scope5/1, [Outside_East_West]
  [Horizontal_Length_South] -> Subsystem/6(Characteristic_length_(m) L)
  Multiport Switch2/1 -> Fcn1/1, [Ambient_Temp_degC], To Workspace/1, Scope32/1
  Clock/1 -> Seoul_Seoul_Temp_(degC) 20200701_to_20200731/1, Seoul_under_30cm_ground_temperature_(degC) 20200901_to_20200930/1, Seoul_under_30cm_ground_temperature_(degC) 20200801_to_20200831/1, Seoul_under_30cm_ground_temperature_(degC) 20200701_to_20200731/1, Seoul_ambient_water_vapor_pressure_(hPa) 20200701_to_20200731/1, Seoul_ambient_water_vapor_pressure_(hPa) 20200801_to_20200831/1, Seoul_ambient_water_vapor_pressure_(hPa) 20200901_to_20200930/1, Seoul_Seoul_Temp_(degC) 20200801_to_20200831/1, Seoul_Seoul_Temp_(degC) 20200901_to_20200930/1, Seoul_Solar_heat_flux_(W/m2) 20200701_to_20200731/1, Seoul_Solar_heat_flux_(W/m2) 20200801_to_20200831/1, Air_wind_speed_(m/s) _of_Air_temperature_(degC)08/1, Air_wind_speed_(m/s) _of_Time/1, Air_wind_speed_(m/s) _of_Air_temperature_(degC)09/1, Seoul_Solar_heat_flux_(W/m2) 20200901_to_20200930/1
  [Ambient_Temp_degC] -> Air_density_(kg/m3) _of_Air_temperature_(degC)/1
  [Ambient_Temp_degC] -> Air_dynamic_viscosity_(Pa s) _of_Air_temperature_(degC)/1
  [Ambient_Temp_degC] -> Air_Prandtl_number_(-) _of_Air_temperature_(degC)/1
  [Ambient_Temp_degC] -> Air_Thermal_conductivity_(W/mK) _of_Air_temperature_(degC)/1
  [Ambient_Temp_K] -> South_Wall_Block/1(Ambient_temperature_[K])
  [Ambient_Temp_K] -> East_Wall_Block/1(Ambient_temperature_[K])
  [Ambient_air_density] -> Subsystem/1(Density)
  [Wind_Speed] -> Subsystem/2(Wind speed (m/s))
  [Ambient_air_dynamic_viscosity] -> Subsystem/3(Dynamic viscosity)
  [Ambient_air_Prandtl_number] -> Subsystem/4(Ptandtl number)
  [Ambient_air_thermal_conductivity] -> Subsystem/5(Air Thermal conductivity(W/mK))
  [Ambient_air_thermal_conductivity] -> Subsystem1/5(Air Thermal conductivity(W/mK))
  [Ambient_air_Prandtl_number] -> Subsystem1/4(Ptandtl number)
  [Ambient_air_dynamic_viscosity] -> Subsystem1/3(Dynamic viscosity)
  [Wind_Speed] -> Subsystem1/2(Wind speed (m/s))
  [Ambient_air_density] -> Subsystem1/1(Density)
  [Horizontal_Length_East] -> Subsystem1/6(Characteristic_length_(m) L)
  South_Wall_Block/4(Q_South_InnerWall_to_InnerAir_[W]) -> [Q_South_InnerWall_to_InnerAir], Scope9/1
  South_Wall_Block/3(South_inner_concrete_wall_temperature_[degC]) -> Scope8/1
  South_Wall_Block/2(South_insulator_temperature_[degC]) -> Scope7/1
  South_Wall_Block/1(South_outer_concrete_wall_temperature_[degC]) -> Scope6/1
  North_Wall_Block/1(North_outer_concrete_wall_temperature_[degC]) -> Scope14/1
  North_Wall_Block/2(North_insulator_temperature_[degC]) -> Scope15/1
  North_Wall_Block/3(North_inner_concrete_wall_temperature_[degC]) -> Scope16/1
  North_Wall_Block/4(Q_North_InnerWall_to_InnerAir_[W]) -> [Q_North_InnerWall_to_InnerAir], Scope17/1
  [Ambient_Temp_K] -> West_Wall_Block/1(Ambient_temperature_[K])
  [Ambient_Temp_K] -> North_Wall_Block/1(Ambient_temperature_[K])
  West_Wall_Block/4(Q_West_InnerWall_to_InnerAir_[W]) -> [Q_West_InnerWall_to_InnerAir], Scope13/1
  West_Wall_Block/3(West_inner_concrete_wall_temperature_[degC]) -> Scope12/1
  West_Wall_Block/2(West_insulator_temperature_[degC]) -> Scope11/1
  West_Wall_Block/1(West_outer_concrete_wall_temperature_[degC]) -> Scope10/1
  Q_total_to_InnerAir_[W]/1 -> Scope33/1, [Q_total_to_InnerAir]
  [Q_East_InnerWall_to_InnerAir] -> Mux4/2
  [Q_South_InnerWall_to_InnerAir] -> Mux4/1
  Mux4/1 -> Q_total_to_InnerAir_[W]/1
  density_window/1 -> [density_window]
  Cp_window/1 -> [Cp_window]
  [Vertical_Length_Window] -> Mux5/2
  [Horizontal_Length_Window] -> Mux5/1
  A=Area_window/1 -> [Area_window]
  Mux5/1 -> A=Area_window/1
  window_depth_[m]/1 -> [window_Depth]
  Window_Block/2(Window_temperature_[degC]) -> Scope18/1
  Window_Block/3(Q_Window_to_InnerAir_[W]) -> [Q_Window_to_InnerAir], Scope19/1
  Window_Block/4(Q_solar_to_InnerAir_[W]) -> [Q_solar_to_InnerAir], Scope20/1
  Window_Block/1(Window_temperature_[K]) -> Terminator/1
  [Ambient_Temp_K] -> Window_Block/1(Ambient_temperature_[K])
  "k_soil Soil Frank P. Incropera and David P. DeWitt, \"Fundamentals of Heat and Mass Transfer\", (1996), FOURTH EDITION, pg. 838"/1 -> [k_soil]
  Under_30cm_soil_Depth_[m]/1 -> [Under_30cm_soil_Depth]
  Mux6/1 -> A=Area_floor/1
  A=Area_floor/1 -> [Area_floor]
  [Horizontal_Length_South] -> Mux6/1
  [Horizontal_Length_East] -> Mux6/2
  Floorl_Block/1(Floor_insulator_temperature_[degC]) -> Scope21/1
  Floorl_Block/2(Floor_inner_wall_temperature_[degC]) -> Scope22/1
  Floorl_Block/3(Q_floor_to_InnerAir_[W]) -> [Q_floor_to_InnerAir], Scope23/1
  [Under_30cm_soil_temperature_K] -> Floorl_Block/1(Under_30cm_soil_temperature_[K])
  Seoul_under_30cm_ground_temperature_(degC) 20200701_to_20200731/1 -> Multiport Switch1/2
  [Q_North_InnerWall_to_InnerAir] -> Mux4/3
  [Q_West_InnerWall_to_InnerAir] -> Scope31/1, Mux4/4
  [Q_solar_to_InnerAir] -> Gain/1
  [Q_Window_to_InnerAir] -> Scope30/1, Mux4/5
  [Q_floor_to_InnerAir] -> Scope28/1, Mux4/7
  AC_evaporator_vertical_length_[m]/1 -> [Vertical_Length_AC_evaporator]
  [Vertical_Length_South] -> Mux7/2
  [Area_floor] -> Mux7/1
  Mux7/1 -> Volume/1
  Volume/1 -> [Volume_room]
  Product/1 -> Scope27/1, Mux4/8
  Product1/1 -> Scope26/1, Mux4/9
  AC_ON/1 -> Product1/2, Product/2, Blower_and_InnerAir_Block/7(AC_ON)
  [AC_outlet_Q] -> Product/1
  [Blower_Q] -> Product1/1
  Blower_and_InnerAir_Block/2(InnerAir_temperature_[degC]) -> InnerAir_temperature_[degC]/1, Scope24/1
  Blower_and_InnerAir_Block/1(InnerAir_temperature_[K]) -> InnerAir_temperature_[K]/1, [InnerAir_Temperature], Scope25/1
  [InnerAir_Temperature] -> South_Wall_Block/2(Inner_air_temperature_[K])
  [InnerAir_Temperature] -> East_Wall_Block/2(Inner_air_temperature_[K])
  [InnerAir_Temperature] -> North_Wall_Block/2(Inner_air_temperature_[K])
  [InnerAir_Temperature] -> West_Wall_Block/2(Inner_air_temperature_[K])
  [InnerAir_Temperature] -> Window_Block/2(Inner_air_temperature_[K])
  [InnerAir_Temperature] -> Floorl_Block/2(Inner_air_temperature_[K])
  [Ambient_Temp_K] -> Blower_and_InnerAir_Block/3(Ambient_temperature_[K]1)
  [Ambient_Water_Vapor_Pressure] -> Blower_and_InnerAir_Block/4(Ambient_water_vapor_pressure_[Pa])
  Infiltration_[L/hr]/1 -> "[L] to [m3]"/1
  "[1/hr] to [1/s]"/1 -> [Infiltration]
  "[L] to [m3]"/1 -> "[1/hr] to [1/s]"/1
  Ventilation_[L/hr]/1 -> "[L] to [m3]2"/1
  "[1/hr] to [1/s]2"/1 -> [Ventilation]
  "[L] to [m3]2"/1 -> "[1/hr] to [1/s]2"/1
  [Ventilation] -> Blower_and_InnerAir_Block/2(Ventilation_[m3/s])
  [Infiltration] -> Blower_and_InnerAir_Block/1(Infiltration_[m3/s])
  AC_blower_Volume_flow_rate_[m3/s]/1 -> [Blower_Volume_Flow_Rate]
  [Blower_Volume_Flow_Rate] -> Blower_and_InnerAir_Block/5(Blower_volume_flow_rate_[m3/s])
  Q_AC_cooling_[W]/1 -> Blower_and_InnerAir_Block/6(Q_AC_cooling_[W])
  Multiport Switch3/1 -> [solar_heat_flux], To Workspace1/1
  20200901_to_20200930/1 -> Manual Switch2/2
  20200801_to_20200831/1 -> Manual Switch2/1
  20200701_to_20200731/1 -> Manual Switch1/1
  Manual Switch2/1 -> Manual Switch1/2
  Manual Switch1/1 -> Multiport Switch2/1, Multiport Switch3/1, Multiport Switch4/1, Multiport Switch/1, Multiport Switch1/1
  Seoul_ambient_water_vapor_pressure_(hPa) 20200701_to_20200731/1 -> Multiport Switch/2
  Seoul_ambient_water_vapor_pressure_(hPa) 20200801_to_20200831/1 -> Multiport Switch/3
  Seoul_ambient_water_vapor_pressure_(hPa) 20200901_to_20200930/1 -> Multiport Switch/4
  Multiport Switch/1 -> "[hPa] to [Pa]"/1
  Multiport Switch1/1 -> Fcn2/1
  Seoul_under_30cm_ground_temperature_(degC) 20200801_to_20200831/1 -> Multiport Switch1/3
  Seoul_under_30cm_ground_temperature_(degC) 20200901_to_20200930/1 -> Multiport Switch1/4
  Seoul_Seoul_Temp_(degC) 20200701_to_20200731/1 -> Multiport Switch2/2
  Seoul_Seoul_Temp_(degC) 20200801_to_20200831/1 -> Multiport Switch2/3
  Seoul_Seoul_Temp_(degC) 20200901_to_20200930/1 -> Multiport Switch2/4
  Seoul_Solar_heat_flux_(W/m2) 20200701_to_20200731/1 -> Multiport Switch3/2
  Seoul_Solar_heat_flux_(W/m2) 20200801_to_20200831/1 -> Multiport Switch3/3
  Seoul_Solar_heat_flux_(W/m2) 20200901_to_20200930/1 -> Multiport Switch3/4
  Air_wind_speed_(m/s) _of_Time/1 -> Multiport Switch4/2
  Air_wind_speed_(m/s) _of_Air_temperature_(degC)08/1 -> Multiport Switch4/3
  Air_wind_speed_(m/s) _of_Air_temperature_(degC)09/1 -> Multiport Switch4/4
  window_transmitivity_[-]/1 -> [transmitivity_window]
  Initial_InnerAir_Temp_[K]/1 -> [Initial_inner_air_Temp]
  Gain/1 -> Scope29/1, Mux4/6
  Seoul_ambient_water_vapor_pressure_(hPa) 20200701_to_1/1 -> "[hPa] to [Pa]1"/1
  Seoul_under_30cm_ground_temperature_(degC) 20200701_to_1/1 -> Fcn3/1
  Clock1/1 -> Seoul_Seoul_Temp_(degC) 20200701_to_1/1, Seoul_Solar_heat_flux_(W/m2) 20200701_to_1/1, Air_wind_speed_(m/s) _of_Air_temperature_(degC)1/1, Shadow(-) _of_Time(s)/1, Seoul_under_30cm_ground_temperature_(degC) 20200701_to_1/1, Seoul_ambient_water_vapor_pressure_(hPa) 20200701_to_1/1
  Seoul_Seoul_Temp_(degC) 20200701_to_1/1 -> Ambient_Temp_degC1/1, Fcn4/1
  Shadow(-) _of_Time(s)/1 -> [solar_angle_East_to_West]
  Fcn4/1 -> Ambient_Temp_K1/1
  Seoul_Solar_heat_flux_(W/m2) 20200701_to_1/1 -> solar_heat_flux1/1
  Constant6/1 -> Ambient_Temp_degC2/1, Fcn5/1
  Constant8/1 -> Q_total_to_InnerAir1/1
  Fcn5/1 -> Ambient_Temp_K2/1
  Constant7/1 -> solar_heat_flux2/1
  "[hPa] to [Pa]"/1 -> [Ambient_Water_Vapor_Pressure]
  "[hPa] to [Pa]1"/1 -> Ambient_Water_Vapor_Pressure/1
  Fcn2/1 -> [Under_30cm_soil_temperature_K]
  Fcn3/1 -> Under_30cm_soil_temperature_K/1
  Fcn1/1 -> [Ambient_Temp_K]
  Multiport Switch4/1 -> [Wind_Speed]
  Air_wind_speed_(m/s) _of_Air_temperature_(degC)1/1 -> Wind_Speed/1
  Constant5/1 -> [absorptivity_inner_wall_South]
  Constant4/1 -> [absorptivity_inner_wall_East]
  Constant3/1 -> [absorptivity_inner_wall_North]
  Constant2/1 -> [absorptivity_inner_wall_West]
  Constant1/1 -> [absorptivity_inner_floor]
  Constant/1 -> [absoptivity_wall]
  window_absorptivity_[-]/1 -> [absorptivity_window]
  "Inside_convection_heat_coefficient_H_(summer) [Kreider J. F. et al., pp.264] [Kreider, J. F., Curtiss, P. S., & Rabl, A. (2009). Heating and cooling of buildings: design for efficiency. CRC Press.]"/1 -> Gain1/1
  Gain1/1 -> [Inside]

== system building_HVAC_V00_027_AI_2019b/AC_Block/On//Off_control_block ==
  Desired_value : Inport
  Actual_value : Inport  Port=2
  Constant : Constant  Value=0
  Constant1 : Constant
  Display : Display
  Memory : Memory  InheritSampleTime=on
  Relational Operator : RelationalOperator  Operator=>  OutDataTypeStr=boolean  RndMeth=Simplest
  Relational Operator1 : RelationalOperator  Operator=<  OutDataTypeStr=boolean  RndMeth=Simplest
  Switch : Switch  Criteria=u2 > Threshold
  Switch1 : Switch  Criteria=u2 > Threshold
  error1 : Sum  Inputs=+-
  error2 : Sum
  On/Off_output_[0,1] : Outport  VectorParamsAs1DForOutWhenUnconnected=off
  wires:
  Desired_value/1 -> error2/1, error1/1
  [HYT] -> error2/2, error1/2
  Actual_value/1 -> Relational Operator1/2, Relational Operator/2
  error1/1 -> Relational Operator/1
  error2/1 -> Relational Operator1/1
  Relational Operator/1 -> Switch/2
  Relational Operator1/1 -> Switch1/2
  Constant/1 -> Switch/1
  Constant1/1 -> Switch1/1
  Switch1/1 -> Switch/3
  Switch/1 -> Memory/1, On/Off_output_[0,1]/1, Display/1
  Memory/1 -> Switch1/3

== system building_HVAC_V00_027_AI_2019b/AC_Block/PI_control_block1 ==
  Desired_value : Inport
  Actual_value : Inport  Port=2
  0_to_1 : Saturate  UpperLimit=1  LowerLimit=0
  Add1 : Sum
  Constant : Constant  Value=0
  Constant1 : Constant  Value=0
  Discreate_integral1 : DiscreteIntegrator  SampleTime=-1  ICPrevOutput=DiscIntNeverNeededParam  ICPrevScaledInput=DiscIntNeverNeededParam
  Display : Display
  Divide : Product  Inputs=**
  Divide2 : Product  Inputs=**
  Fuzzy Logic Controller : fuzblock/Fuzzy Logic  Controller  FIS=SugenoFuzzy  OutputSampleNumber=101  DataType=double  FuzzifiedInputs=off  RuleFiringStrengths=off  RuleOutputs=off  AggregatedOutputs=off  SimulateUsing=Interpreted execution  OutOfRangeInputValueMessage=warning  NoRuleFiredMessage=warning  EmptyOutputFuzzySetMessage=warning
  Manual Switch : ManualSwitch
  Manual Switch1 : ManualSwitch
  Mux : Mux  Inputs=2
  Plus : Sum
  Plus1 : Sum  Inputs=+-
  Scope{,1..8} (9 alike) : Scope
  Switch1 : Switch  Criteria=u2 > Threshold
  Switch2 : Switch  Criteria=u2 > Threshold
  error : Sum  Inputs=+-
  error1 : Sum  Inputs=+-
  PI_output_[0,1] : Outport  VectorParamsAs1DForOutWhenUnconnected=off
  wires:
  Desired_value/1 -> error/2, error1/1, Mux/1, Plus1/2
  Actual_value/1 -> Plus1/1, error/1, error1/2
  Add1/1 -> Scope5/1, 0_to_1/1
  0_to_1/1 -> Scope/1, PI_output_[0,1]/1, Display/1
  Discreate_integral1/1 -> Scope2/1, Divide2/2
  [I_value] -> Divide2/1
  [P_value] -> Divide/2
  Divide2/1 -> Add1/1, Scope3/1
  Divide/1 -> Add1/2, Scope4/1
  error/1 -> Switch1/1, Switch1/2
  Constant/1 -> Switch1/3
  error1/1 -> Manual Switch/1
  Switch1/1 -> Manual Switch/2
  Fuzzy Logic Controller/1 -> Scope7/1, Plus/1
  Plus/1 -> Scope6/1, Switch2/2, Switch2/1
  Mux/1 -> Fuzzy Logic Controller/1, Scope8/1
  Plus1/1 -> Mux/2, Plus/2
  Constant1/1 -> Switch2/3
  Manual Switch/1 -> Manual Switch1/2
  Switch2/1 -> Manual Switch1/1
  Manual Switch1/1 -> Divide/1, Discreate_integral1/1, Scope1/1

== system building_HVAC_V00_027_AI_2019b/AC_Block/PI_control_block2 ==
  Desired_value : Inport
  Actual_value : Inport  Port=2
  0_to_1 : Saturate  UpperLimit=1  LowerLimit=0
  Add1 : Sum
  Discreate_integral1 : DiscreteIntegrator  SampleTime=-1  ICPrevOutput=DiscIntNeverNeededParam  ICPrevScaledInput=DiscIntNeverNeededParam
  Display : Display
  Divide : Product  Inputs=**
  Divide2 : Product  Inputs=**
  error : Sum  Inputs=+-
  PI_output_[0,1] : Outport  VectorParamsAs1DForOutWhenUnconnected=off
  wires:
  Divide/1 -> Add1/2
  Divide2/1 -> Add1/1
  [P_value_Variable_speed] -> Divide/2
  [I_value_Variable_speed] -> Divide2/1
  Discreate_integral1/1 -> Divide2/2
  0_to_1/1 -> Display/1, PI_output_[0,1]/1
  Add1/1 -> 0_to_1/1
  Actual_value/1 -> error/2
  error/1 -> Discreate_integral1/1, Divide/1
  Desired_value/1 -> error/1
